simulink subsystem "VCM_main"  (R2021b)
settings: Solver=VariableStepAuto  StartTime=0.0  StopTime=10.0  RelTol=1e-3
values from neighbouring files (symbols this model uses):
  g = 9.80665    [VehicleParamsFEM20_Gear17.m]
  gear_f = 14.45    [VehicleParamsFEM20_Gear17.m]
  gear_r = 14.45    [VehicleParamsFEM20_Gear17.m]
  Iwf = 0.2    [VehicleParamsFEM20_Gear17.m]
  Rwf = 18*(25.4/1000)/2    (= 0.2286)    [VehicleParamsFEM20_Gear17.m]
libraries: simulink x46, dspswit3 x1, slpidlib x1
(part 3 of 5)

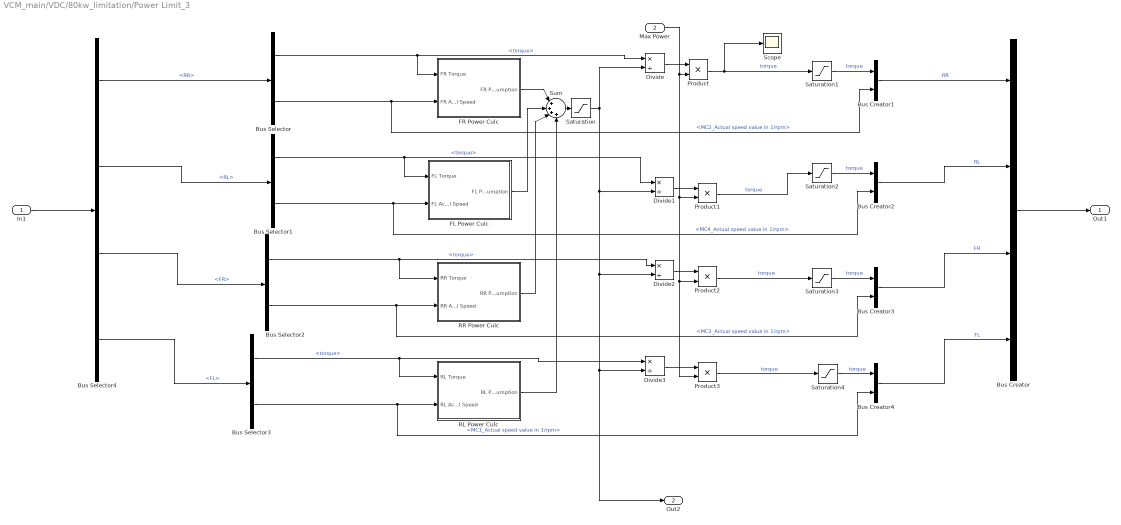
== system VCM_main/VDC/80kw_limitation/Power Limit_3 ==
  In1 : Inport
  Max Power : Inport  Port=2
  Bus Creator : BusCreator  Inputs=4
  Bus Creator{1..4} (4 alike) : BusCreator  Inputs=2
  Bus Selector : BusSelector  OutputSignals=torque,MC2_Actual speed value in 1/rpm
  Bus Selector1 : BusSelector  OutputSignals=torque,MC4_Actual speed value in 1/rpm
  Bus Selector2 : BusSelector  OutputSignals=torque,MC3_Actual speed value in 1/rpm
  Bus Selector3 : BusSelector  OutputSignals=torque,MC1_Actual speed value in 1/rpm
  Bus Selector4 : BusSelector  OutputSignals=RR,RL,FR,FL
  Divide{,1..3} (4 alike) : Product  Inputs=*/
  FL Power Culc : Subsystem
  FR Power Culc : Subsystem
  Product{,1..3} (4 alike) : Product
  RL Power Culc : Subsystem
  RR Power Culc : Subsystem
  Saturation : Saturate  UpperLimit=inf  LowerLimit=1
  Saturation{1..4} (4 alike) : Saturate  UpperLimit=21  LowerLimit=-21
  Scope : Scope
  Sum : Sum  Inputs=|++++
  Out1 : Outport  VectorParamsAs1DForOutWhenUnconnected=off
  Out2 : Outport  Port=2  VectorParamsAs1DForOutWhenUnconnected=off
  wires:
  Saturation4/1 -> Bus Creator4/1  "torque"
  Saturation3/1 -> Bus Creator3/1  "torque"
  Saturation2/1 -> Bus Creator2/1  "torque"
  Saturation1/1 -> Bus Creator1/1  "torque"
  Product1/1 -> Saturation2/1  "torque"
  Sum/1 -> Saturation/1
  Bus Creator4/1 -> Bus Creator/4  "FL"
  Product3/1 -> Saturation4/1  "torque"
  Bus Creator3/1 -> Bus Creator/3  "FR"
  Product2/1 -> Saturation3/1  "torque"
  Bus Creator2/1 -> Bus Creator/2  "RL"
  Bus Creator1/1 -> Bus Creator/1  "RR"
  Product/1 -> Saturation1/1, Scope/1  "torque"
  Bus Selector2/1 -> Divide2/1, RR Power Culc/1(RR Torque)  "<torque>"
  Bus Selector/1 -> FR Power Culc/1(FR Torque), Divide/1  "<torque>"
  Bus Selector1/2 -> Bus Creator2/2, FL Power Culc/2(FL Actual Speed)  "<MC4_Actual speed value in 1/rpm>"
  Bus Selector4/2 -> Bus Selector1/1  "<RL>"
  Saturation/1 -> Divide/2, Divide1/2, Divide2/2, Divide3/2, Out2/1
  Bus Selector3/1 -> RL Power Culc/1(RL Torque), Divide3/1  "<torque>"
  Bus Selector2/2 -> Bus Creator3/2, RR Power Culc/2(RR Actual Speed)  "<MC3_Actual speed value in 1/rpm>"
  Bus Selector1/1 -> FL Power Culc/1(FL Torque), Divide1/1  "<torque>"
  Bus Selector3/2 -> Bus Creator4/2, RL Power Culc/2(RL Actual Speed)  "<MC1_Actual speed value in 1/rpm>"
  RR Power Culc/1(RR Power Consumption) -> Sum/3
  RL Power Culc/1(RL Power Consumption) -> Sum/4
  Bus Selector4/1 -> Bus Selector/1  "<RR>"
  Divide/1 -> Product/1
  Divide1/1 -> Product1/1
  Bus Selector/2 -> Bus Creator1/2, FR Power Culc/2(FR Actual Speed)  "<MC2_Actual speed value in 1/rpm>"
  In1/1 -> Bus Selector4/1
  FR Power Culc/1(FR Power Consumption) -> Sum/1
  FL Power Culc/1(FL Power Consumption) -> Sum/2
  Bus Creator/1 -> Out1/1
  Bus Selector4/4 -> Bus Selector3/1  "<FL>"
  Bus Selector4/3 -> Bus Selector2/1  "<FR>"
  Divide3/1 -> Product3/1
  Divide2/1 -> Product2/1
  Max Power/1 -> Product/2, Product1/2, Product2/2, Product3/2

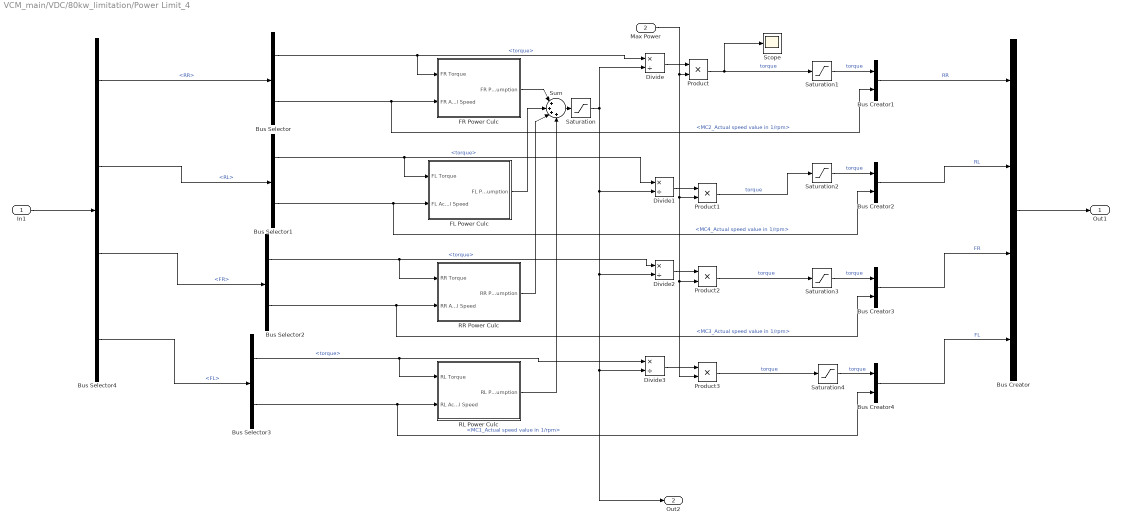
== system VCM_main/VDC/80kw_limitation/Power Limit_4 ==
  In1 : Inport
  Max Power : Inport  Port=2
  Bus Creator : BusCreator  Inputs=4
  Bus Creator{1..4} (4 alike) : BusCreator  Inputs=2
  Bus Selector : BusSelector  OutputSignals=torque,MC2_Actual speed value in 1/rpm
  Bus Selector1 : BusSelector  OutputSignals=torque,MC4_Actual speed value in 1/rpm
  Bus Selector2 : BusSelector  OutputSignals=torque,MC3_Actual speed value in 1/rpm
  Bus Selector3 : BusSelector  OutputSignals=torque,MC1_Actual speed value in 1/rpm
  Bus Selector4 : BusSelector  OutputSignals=RR,RL,FR,FL
  Divide{,1..3} (4 alike) : Product  Inputs=*/
  FL Power Culc : Subsystem
  FR Power Culc : Subsystem
  Product{,1..3} (4 alike) : Product
  RL Power Culc : Subsystem
  RR Power Culc : Subsystem
  Saturation : Saturate  UpperLimit=inf  LowerLimit=1
  Saturation{1..4} (4 alike) : Saturate  UpperLimit=21  LowerLimit=-21
  Scope : Scope
  Sum : Sum  Inputs=|++++
  Out1 : Outport  VectorParamsAs1DForOutWhenUnconnected=off
  Out2 : Outport  Port=2  VectorParamsAs1DForOutWhenUnconnected=off
  wires:
  Max Power/1 -> Product3/2, Product2/2, Product1/2, Product/2
  Divide2/1 -> Product2/1
  Divide3/1 -> Product3/1
  Bus Selector4/3 -> Bus Selector2/1  "<FR>"
  Bus Selector4/4 -> Bus Selector3/1  "<FL>"
  Bus Creator/1 -> Out1/1
  FL Power Culc/1(FL Power Consumption) -> Sum/2
  FR Power Culc/1(FR Power Consumption) -> Sum/1
  In1/1 -> Bus Selector4/1
  Bus Selector/2 -> FR Power Culc/2(FR Actual Speed), Bus Creator1/2  "<MC2_Actual speed value in 1/rpm>"
  Divide1/1 -> Product1/1
  Divide/1 -> Product/1
  Bus Selector4/1 -> Bus Selector/1  "<RR>"
  RL Power Culc/1(RL Power Consumption) -> Sum/4
  RR Power Culc/1(RR Power Consumption) -> Sum/3
  Bus Selector3/2 -> RL Power Culc/2(RL Actual Speed), Bus Creator4/2  "<MC1_Actual speed value in 1/rpm>"
  Bus Selector1/1 -> Divide1/1, FL Power Culc/1(FL Torque)  "<torque>"
  Bus Selector2/2 -> RR Power Culc/2(RR Actual Speed), Bus Creator3/2  "<MC3_Actual speed value in 1/rpm>"
  Bus Selector3/1 -> Divide3/1, RL Power Culc/1(RL Torque)  "<torque>"
  Saturation/1 -> Divide3/2, Out2/1, Divide2/2, Divide1/2, Divide/2
  Bus Selector4/2 -> Bus Selector1/1  "<RL>"
  Bus Selector1/2 -> FL Power Culc/2(FL Actual Speed), Bus Creator2/2  "<MC4_Actual speed value in 1/rpm>"
  Bus Selector/1 -> Divide/1, FR Power Culc/1(FR Torque)  "<torque>"
  Bus Selector2/1 -> RR Power Culc/1(RR Torque), Divide2/1  "<torque>"
  Product/1 -> Scope/1, Saturation1/1  "torque"
  Bus Creator1/1 -> Bus Creator/1  "RR"
  Bus Creator2/1 -> Bus Creator/2  "RL"
  Product2/1 -> Saturation3/1  "torque"
  Bus Creator3/1 -> Bus Creator/3  "FR"
  Product3/1 -> Saturation4/1  "torque"
  Bus Creator4/1 -> Bus Creator/4  "FL"
  Sum/1 -> Saturation/1
  Product1/1 -> Saturation2/1  "torque"
  Saturation1/1 -> Bus Creator1/1  "torque"
  Saturation2/1 -> Bus Creator2/1  "torque"
  Saturation3/1 -> Bus Creator3/1  "torque"
  Saturation4/1 -> Bus Creator4/1  "torque"

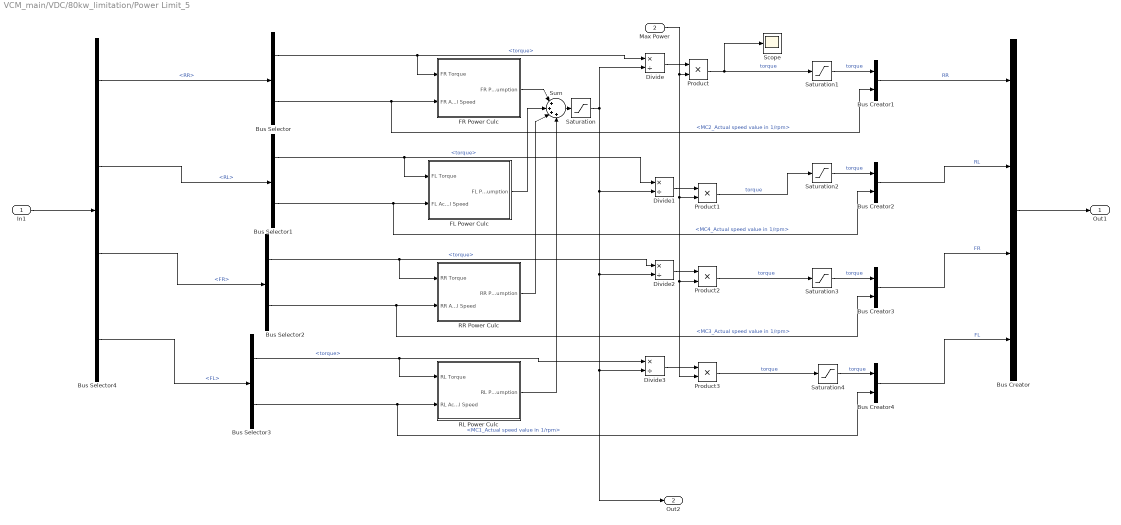
== system VCM_main/VDC/80kw_limitation/Power Limit_5 ==
  In1 : Inport
  Max Power : Inport  Port=2
  Bus Creator : BusCreator  Inputs=4
  Bus Creator{1..4} (4 alike) : BusCreator  Inputs=2
  Bus Selector : BusSelector  OutputSignals=torque,MC2_Actual speed value in 1/rpm
  Bus Selector1 : BusSelector  OutputSignals=torque,MC4_Actual speed value in 1/rpm
  Bus Selector2 : BusSelector  OutputSignals=torque,MC3_Actual speed value in 1/rpm
  Bus Selector3 : BusSelector  OutputSignals=torque,MC1_Actual speed value in 1/rpm
  Bus Selector4 : BusSelector  OutputSignals=RR,RL,FR,FL
  Divide{,1..3} (4 alike) : Product  Inputs=*/
  FL Power Culc : Subsystem
  FR Power Culc : Subsystem
  Product{,1..3} (4 alike) : Product
  RL Power Culc : Subsystem
  RR Power Culc : Subsystem
  Saturation : Saturate  UpperLimit=inf  LowerLimit=1
  Saturation{1..4} (4 alike) : Saturate  UpperLimit=21  LowerLimit=-21
  Scope : Scope
  Sum : Sum  Inputs=|++++
  Out1 : Outport  VectorParamsAs1DForOutWhenUnconnected=off
  Out2 : Outport  Port=2  VectorParamsAs1DForOutWhenUnconnected=off
  wires:
  Saturation4/1 -> Bus Creator4/1  "torque"
  Saturation3/1 -> Bus Creator3/1  "torque"
  Saturation2/1 -> Bus Creator2/1  "torque"
  Saturation1/1 -> Bus Creator1/1  "torque"
  Product1/1 -> Saturation2/1  "torque"
  Sum/1 -> Saturation/1
  Bus Creator4/1 -> Bus Creator/4  "FL"
  Product3/1 -> Saturation4/1  "torque"
  Bus Creator3/1 -> Bus Creator/3  "FR"
  Product2/1 -> Saturation3/1  "torque"
  Bus Creator2/1 -> Bus Creator/2  "RL"
  Bus Creator1/1 -> Bus Creator/1  "RR"
  Product/1 -> Saturation1/1, Scope/1  "torque"
  Bus Selector2/1 -> Divide2/1, RR Power Culc/1(RR Torque)  "<torque>"
  Bus Selector/1 -> FR Power Culc/1(FR Torque), Divide/1  "<torque>"
  Bus Selector1/2 -> Bus Creator2/2, FL Power Culc/2(FL Actual Speed)  "<MC4_Actual speed value in 1/rpm>"
  Bus Selector4/2 -> Bus Selector1/1  "<RL>"
  Saturation/1 -> Divide/2, Divide1/2, Divide2/2, Divide3/2, Out2/1
  Bus Selector3/1 -> RL Power Culc/1(RL Torque), Divide3/1  "<torque>"
  Bus Selector2/2 -> Bus Creator3/2, RR Power Culc/2(RR Actual Speed)  "<MC3_Actual speed value in 1/rpm>"
  Bus Selector1/1 -> FL Power Culc/1(FL Torque), Divide1/1  "<torque>"
  Bus Selector3/2 -> Bus Creator4/2, RL Power Culc/2(RL Actual Speed)  "<MC1_Actual speed value in 1/rpm>"
  RR Power Culc/1(RR Power Consumption) -> Sum/3
  RL Power Culc/1(RL Power Consumption) -> Sum/4
  Bus Selector4/1 -> Bus Selector/1  "<RR>"
  Divide/1 -> Product/1
  Divide1/1 -> Product1/1
  Bus Selector/2 -> Bus Creator1/2, FR Power Culc/2(FR Actual Speed)  "<MC2_Actual speed value in 1/rpm>"
  In1/1 -> Bus Selector4/1
  FR Power Culc/1(FR Power Consumption) -> Sum/1
  FL Power Culc/1(FL Power Consumption) -> Sum/2
  Bus Creator/1 -> Out1/1
  Bus Selector4/4 -> Bus Selector3/1  "<FL>"
  Bus Selector4/3 -> Bus Selector2/1  "<FR>"
  Divide3/1 -> Product3/1
  Divide2/1 -> Product2/1
  Max Power/1 -> Product/2, Product1/2, Product2/2, Product3/2

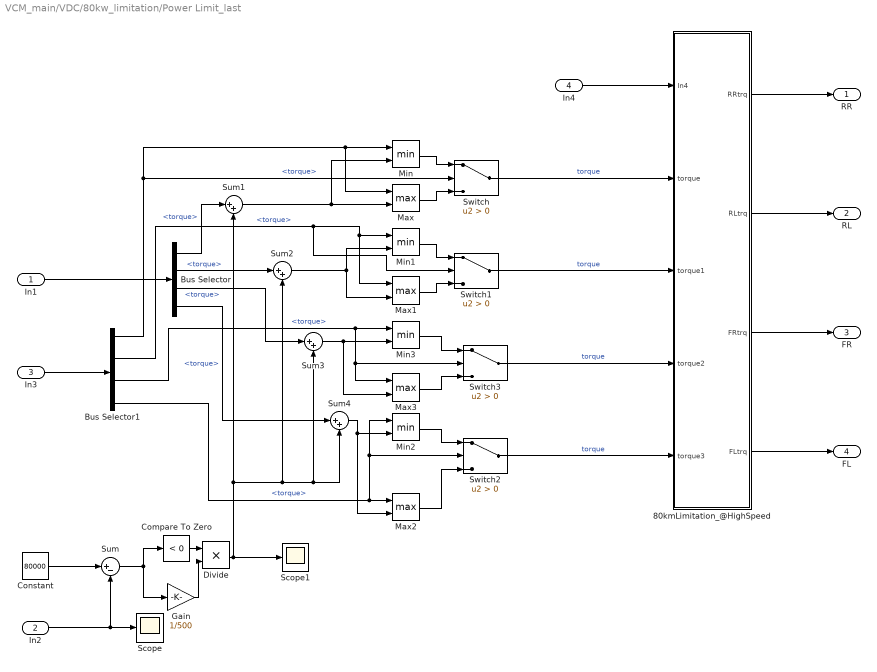
== system VCM_main/VDC/80kw_limitation/Power Limit_last ==
  In1 : Inport
  In2 : Inport  Port=2
  In3 : Inport  Port=3
  In4 : Inport  Port=4
  80kmLimitation_@HighSpeed : Subsystem
  Bus Selector : BusSelector  OutputSignals=RR.torque,RL.torque,FR.torque,FL.torque
  Bus Selector1 : BusSelector  OutputSignals=RR.torque,RL.torque,FR.torque,FL.torque
  Compare To Zero : simulink/Logic and Bit Operations/Compare To Zero  relop=<  OutDataTypeStr=boolean
  Constant : Constant  Value=80000
  Divide : Product  Inputs=**
  Gain : Gain  Gain=1/500
  Max{,1..3} (4 alike) : MinMax  Function=max  Inputs=2
  Min{,1..3} (4 alike) : MinMax  Inputs=2
  Scope : Scope
  Scope1 : Scope
  Sum : Sum  Inputs=|+-
  Sum{1..4} (4 alike) : Sum  Inputs=|++
  Switch{,1..3} (4 alike) : Switch  Criteria=u2 > Threshold
  RR : Outport  VectorParamsAs1DForOutWhenUnconnected=off
  RL : Outport  Port=2  VectorParamsAs1DForOutWhenUnconnected=off
  FR : Outport  Port=3  VectorParamsAs1DForOutWhenUnconnected=off
  FL : Outport  Port=4  VectorParamsAs1DForOutWhenUnconnected=off
  wires:
  Gain/1 -> Divide/2
  Compare To Zero/1 -> Divide/1
  80kmLimitation_@HighSpeed/4(FLtrq) -> FL/1
  80kmLimitation_@HighSpeed/2(RLtrq) -> RL/1
  80kmLimitation_@HighSpeed/3(FRtrq) -> FR/1
  80kmLimitation_@HighSpeed/1(RRtrq) -> RR/1
  Switch2/1 -> 80kmLimitation_@HighSpeed/5(torque3)  "torque"
  Switch3/1 -> 80kmLimitation_@HighSpeed/4(torque2)  "torque"
  Switch1/1 -> 80kmLimitation_@HighSpeed/3(torque1)  "torque"
  Switch/1 -> 80kmLimitation_@HighSpeed/2(torque)  "torque"
  In4/1 -> 80kmLimitation_@HighSpeed/1(In4)
  Max3/1 -> Switch3/3
  Min3/1 -> Switch3/1
  Max2/1 -> Switch2/3
  Min2/1 -> Switch2/1
  Max1/1 -> Switch1/3
  Min1/1 -> Switch1/1
  Max/1 -> Switch/3
  Min/1 -> Switch/1
  Bus Selector1/4 -> Max2/1, Switch2/2, Min2/1  "<torque>"
  Sum4/1 -> Min2/2, Max2/2
  Bus Selector1/3 -> Min3/1, Switch3/2, Max3/1  "<torque>"
  Sum3/1 -> Min3/2, Max3/2
  Bus Selector1/2 -> Min1/1, Max1/1, Switch1/2  "<torque>"
  Sum2/1 -> Min1/2, Max1/2
  Bus Selector1/1 -> Max/1, Min/1, Switch/2  "<torque>"
  Sum1/1 -> Min/2, Max/2
  In3/1 -> Bus Selector1/1
  Bus Selector/4 -> Sum4/1  "<torque>"
  Bus Selector/3 -> Sum3/1  "<torque>"
  Bus Selector/2 -> Sum2/1  "<torque>"
  Divide/1 -> Scope1/1, Sum3/2, Sum4/2, Sum2/2, Sum1/2
  Bus Selector/1 -> Sum1/1  "<torque>"
  In1/1 -> Bus Selector/1
  Sum/1 -> Gain/1, Compare To Zero/1
  In2/1 -> Scope/1, Sum/2
  Constant/1 -> Sum/1

== system VCM_main/VDC/80kw_limitation/Subsystem ==
  In1 : Inport
  RR : Inport  Port=2
  RL : Inport  Port=3
  FR : Inport  Port=4
  FL : Inport  Port=5
  Bus Creator : BusCreator  Inputs=4
  Bus Selector : BusSelector  OutputSignals=RR.torque,RL.torque,FR.torque,FL.torque
  Switch{,1..3} (4 alike) : Switch  Criteria=u2 > Threshold  Threshold=0.5
  Out1 : Outport  VectorParamsAs1DForOutWhenUnconnected=off
  wires:
  RL/1 -> Switch1/1
  RR/1 -> Switch/1
  In1/1 -> Bus Selector/1
  FR/1 -> Switch2/1
  Bus Selector/2 -> Switch1/3  "<torque>"
  Switch3/1 -> Bus Creator/4  "FLtorque"
  Switch1/1 -> Bus Creator/2  "RLtorque"
  Bus Creator/1 -> Out1/1
  Bus Selector/4 -> Switch3/3  "<torque>"
  Switch/1 -> Bus Creator/1  "RRtorque"
  FL/1 -> Switch3/1
  Switch2/1 -> Bus Creator/3  "FRtorque"
  Bus Selector/1 -> Switch/3  "<torque>"
  [PowerLimitOn] -> Switch1/2, Switch/2, Switch2/2, Switch3/2
  Bus Selector/3 -> Switch2/3  "<torque>"

== system VCM_main/VDC/DYC/Moment to ΔT ==
  TargetYawMoment : Inport
  Gain12 : Gain  Gain=1/4
  Gain13 : Gain  Gain=1/0.625
  Gain14 : Gain  Gain=1/13.75
  Gain4 : Gain  Gain=18*(25.4/1000)/2
  Saturation : Saturate  UpperLimit=5  LowerLimit=-5
  DYC_deltaTorque : Outport
  wires:
  Saturation/1 -> DYC_deltaTorque/1  "DYC_deltaTorque"
  Gain4/1 -> Saturation/1
  Gain14/1 -> Gain4/1
  Gain12/1 -> Gain13/1
  TargetYawMoment/1 -> Gain12/1
  Gain13/1 -> Gain14/1

== system VCM_main/VDC/DYC/Torque distributor1 ==
  Torque In : Inport
  In2 : Inport  Port=2
  Add : Sum
  Logical Operator : Logic  AllPortsSameDT=off  OutDataTypeStr=boolean
  Switch : Switch  Criteria=u2 > Threshold  Threshold=0.5
  torque : Outport
  wires:
  Logical Operator/1 -> Switch/2
  [All_bQuitInverterOn] -> Logical Operator/2
  Switch/1 -> torque/1
  [DYCOn] -> Logical Operator/1
  In2/1 -> Add/2
  Add/1 -> Switch/1  "torque"
  Torque In/1 -> Add/1, Switch/3

== system VCM_main/VDC/DYC/Torque distributor2 ==
  Torque In : Inport
  In2 : Inport  Port=2
  Add : Sum
  Logical Operator : Logic  AllPortsSameDT=off  OutDataTypeStr=boolean
  Switch : Switch  Criteria=u2 > Threshold  Threshold=0.5
  torque : Outport
  wires:
  Torque In/1 -> Switch/3, Add/1
  Add/1 -> Switch/1  "torque"
  In2/1 -> Add/2
  [DYCOn] -> Logical Operator/1
  Switch/1 -> torque/1
  [All_bQuitInverterOn] -> Logical Operator/2
  Logical Operator/1 -> Switch/2

== system VCM_main/VDC/DYC/Torque distributor3 ==
  Torque In : Inport
  In2 : Inport  Port=2
  Add : Sum
  Logical Operator : Logic  AllPortsSameDT=off  OutDataTypeStr=boolean
  Switch : Switch  Criteria=u2 > Threshold  Threshold=0.5
  torque : Outport
  wires:
  Logical Operator/1 -> Switch/2
  [All_bQuitInverterOn] -> Logical Operator/2
  Switch/1 -> torque/1
  [DYCOn] -> Logical Operator/1
  In2/1 -> Add/2
  Add/1 -> Switch/1  "torque"
  Torque In/1 -> Add/1, Switch/3

== system VCM_main/VDC/DYC/Torque distributor4 ==
  Torque In : Inport
  DYC_deltaTorque : Inport  Port=2
  Add : Sum
  Logical Operator : Logic  AllPortsSameDT=off  OutDataTypeStr=boolean
  Switch : Switch  Criteria=u2 > Threshold  Threshold=0.5
  torque : Outport
  wires:
  Torque In/1 -> Switch/3, Add/1
  Add/1 -> Switch/1  "torque"
  DYC_deltaTorque/1 -> Add/2
  [DYCOn] -> Logical Operator/1
  Switch/1 -> torque/1
  [All_bQuitInverterOn] -> Logical Operator/2
  Logical Operator/1 -> Switch/2

== system VCM_main/VDC/DYC/YawmomentCal ==
  DriverInput : Inport
  Sensor : Inport  Port=2
  Bus Selector1 : BusSelector  OutputSignals=CAN_from_IMU_122.GYRO_Z,CAN_from_IMU_220.ANGLE_SLIP
  Bus Selector2 : BusSelector  OutputSignals=SteerAngle_Actual
  FB : Subsystem
  FF_Gain : Subsystem
  FF_diff_Gain : Subsystem
  Gain : Gain  Gain=300
  Ground : Ground
  Scope : Scope
  Sensor1 : InportShadow  Port=2
  StabilityFactor_ref : Constant  Value=0.00125
  Sum : Sum  Inputs=|++
  Sum1 : Sum  Inputs=|++
  Sum2 : Sum  Inputs=|-+
  Terminator : Terminator
  Terminator1 : Terminator
  Terminator3 : Terminator
  Velocity Clc : Subsystem
  stabilityfactor_noDYC : Constant  Value=0.00604
  δ to r_noDYC : Subsystem
  δ to r_ref : Subsystem
  TargetYawMoment : Outport  VectorParamsAs1DForOutWhenUnconnected=off
  r_ref : Outport  Port=2
  wires:
  Sum1/1 -> Terminator3/1
  FB/1(y) -> Sum1/2
  Ground/1 -> Sum/2
  Bus Selector1/1 -> FB/2(<GYRO_Z>)  "<GYRO_Z>"
  Sum/1 -> Sum1/1
  FF_diff_Gain/1(Out1) -> Terminator/1
  FF_Gain/1(Out1) -> Sum/1
  Velocity Clc/1(v [m/s]) -> δ to r_ref/1(v [m/s]), δ to r_noDYC/1(v [m/s]), FF_Gain/1(v [m/s]), FF_diff_Gain/1(v [m/s])
  Sensor/1 -> Velocity Clc/1(Sensor)
  Bus Selector1/2 -> Terminator1/1  "<ANGLE_SLIP>"
  Sensor1/1 -> Bus Selector1/1
  Sum2/1 -> FF_Gain/2(In1), FF_diff_Gain/2(In2), Scope/1
  Gain/1 -> TargetYawMoment/1  "TargetYawMoment"
  δ to r_noDYC/1(r_noDYC) -> Sum2/1  "r_noDYC"
  stabilityfactor_noDYC/1 -> δ to r_noDYC/2(StabilityFactor)
  Bus Selector2/1 -> δ to r_noDYC/3(SteerAngle), δ to r_ref/3(SteerAngle), Gain/1  "<SteerAngle_Actual>"
  DriverInput/1 -> Bus Selector2/1
  δ to r_ref/1(r_ref) -> Sum2/2, FB/1(r_ref), r_ref/1  "r_ref"
  StabilityFactor_ref/1 -> δ to r_ref/2(StabilityFactor)

== system VCM_main/VDC/Launch/max rpm ==
  Can Inv : Inport
  Bus Selector4 : BusSelector  OutputSignals=MC_11.MC1_Actual speed value in 1/rpm,MC_31.MC3_Actual speed value in 1/rpm,MC_21.MC2_Actual speed value in 1/rpm,MC_41.MC4_Actual speed value in 1/rpm
  Min : MinMax  Function=max  Inputs=4
  max rpm : Outport
  wires:
  Bus Selector4/2 -> Min/2  "<MC3_Actual speed value in 1/rpm>"
  Bus Selector4/3 -> Min/3  "<MC2_Actual speed value in 1/rpm>"
  Bus Selector4/1 -> Min/1  "<MC1_Actual speed value in 1/rpm>"
  Min/1 -> max rpm/1  "max rpm"
  Can Inv/1 -> Bus Selector4/1
  Bus Selector4/4 -> Min/4  "<MC4_Actual speed value in 1/rpm>"

== system VCM_main/VDC/Torque Front//rear distributor Main/Max Torque Limit ==
  note: MAXトルクオーバーしている分だけもう一方に振り直し
  Max Torque : Inport
  torque_front : Inport  Port=2
  torque_rear : Inport  Port=3
  Add10 : Sum  Inputs=-+
  Add11 : Sum
  Add4 : Sum  Inputs=+-
  Add7 : Sum  Inputs=+-
  Add8 : Sum
  Add9 : Sum  Inputs=+-
  Display : Display
  Display5 : Display
  Display6 : Display
  Saturation : Saturate  UpperLimit=inf  LowerLimit=0
  Saturation3 : Saturate  UpperLimit=inf  LowerLimit=0
  torque_front Out : Outport
  torque_rear Out : Outport  Port=2
  wires:
  Max Torque/1 -> Add9/2, Add4/2
  Add11/1 -> torque_rear Out/1
  Add7/1 -> Add11/2
  Add4/1 -> Saturation/1
  Add10/1 -> torque_front Out/1
  Add8/1 -> Add10/2
  torque_rear/1 -> Display6/1, Add7/1, Add4/1
  Add9/1 -> Saturation3/1
  torque_front/1 -> Display5/1, Add8/1, Add9/1
  Saturation3/1 -> Add10/1, Add11/1
  Saturation/1 -> Display/1, Add7/2, Add8/2

== system VCM_main/VDC/Torque Front//rear distributor Main/Min Torque Limit ==
  note: MINトルクオーバーしている分だけもう一方に振り直し
  Min Torque : Inport
  torque_front : Inport  Port=2
  torque_rear : Inport  Port=3
  Add10 : Sum  Inputs=-+
  Add11 : Sum
  Add4 : Sum  Inputs=+-
  Add7 : Sum  Inputs=+-
  Add8 : Sum
  Add9 : Sum  Inputs=+-
  Display{,1..2,5..6} (5 alike) : Display
  Gain : Gain  Gain=-1
  Saturation : Saturate  UpperLimit=0  LowerLimit=-inf
  Saturation3 : Saturate  UpperLimit=0  LowerLimit=-inf
  torque_rear Out : Outport
  torque_front Out : Outport  Port=2
  wires:
  Gain/1 -> Add9/2, Add4/2
  Min Torque/1 -> Gain/1
  Add11/1 -> torque_rear Out/1  "torque_rear"
  Add7/1 -> Add11/2, Display1/1
  Add4/1 -> Saturation/1
  Add10/1 -> torque_front Out/1  "torque_front"
  Add8/1 -> Add10/2
  torque_rear/1 -> Display6/1, Add7/1, Add4/1
  Add9/1 -> Saturation3/1
  torque_front/1 -> Display5/1, Add8/1, Add9/1
  Saturation3/1 -> Add10/1, Add11/1, Display2/1
  Saturation/1 -> Display/1, Add7/2, Add8/2

== system VCM_main/VDC/Torque Front//rear distributor Main/Saturation ==
  u : Inport
  Saturation Dynamic1 : simulink/Discontinuities/Saturation Dynamic  OutMin=[]  OutMax=[]  OutDataTypeStr=Inherit: Same as second input  OutDataType=fixdt(1, 16)  OutScaling=2^-10  DoSatur=off
  y : Outport
  wires:
  u/1 -> Saturation Dynamic1/2
  Saturation Dynamic1/1 -> y/1
  [MinTorque] -> Saturation Dynamic1/3
  [MaxTorque] -> Saturation Dynamic1/1

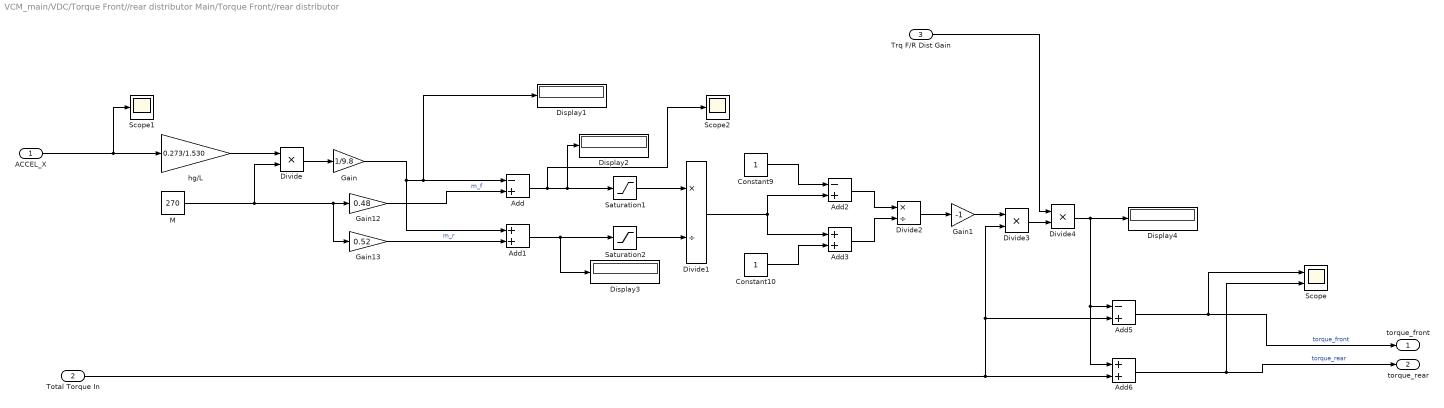
== system VCM_main/VDC/Torque Front//rear distributor Main/Torque Front//rear distributor  ==
  ACCEL_X : Inport
  Total Torque In : Inport  Port=2
  Trq F/R Dist Gain : Inport  Port=3
  Add : Sum  Inputs=-+
  Add1 : Sum
  Add2 : Sum  Inputs=-+
  Add3 : Sum
  Add5 : Sum  Inputs=-+
  Add6 : Sum
  Constant10 : Constant
  Constant9 : Constant
  Display{1..4} (4 alike) : Display
  Divide : Product  Inputs=**
  Divide1 : Product  Inputs=*/
  Divide2 : Product  Inputs=*/
  Divide3 : Product  Inputs=**
  Divide4 : Product  Inputs=**
  Gain : Gain  Gain=1/9.8
  Gain1 : Gain  Gain=-1
  Gain12 : Gain  Gain=0.48
  Gain13 : Gain  Gain=0.52
  M : Constant  Value=270
  Saturation1 : Saturate  UpperLimit=270  LowerLimit=10
  Saturation2 : Saturate  UpperLimit=270  LowerLimit=10
  Scope : Scope  NumInputPorts=2
  Scope1 : Scope
  Scope2 : Scope
  hg/L : Gain  Gain=0.273/1.530
  torque_front : Outport
  torque_rear : Outport  Port=2
  wires:
  Divide/1 -> Gain/1
  Total Torque In/1 -> Divide3/2, Add5/2, Add6/2
  Trq F/R Dist Gain/1 -> Divide4/1
  Divide3/1 -> Divide4/2
  Add5/1 -> torque_front/1, Scope/1  "torque_front"
  Add6/1 -> torque_rear/1, Scope/2  "torque_rear"
  Gain13/1 -> Add1/2  "m_r"
  Saturation1/1 -> Divide1/1
  Add/1 -> Saturation1/1, Display2/1, Scope2/1
  Gain/1 -> Add/1, Display1/1, Add1/1
  Add1/1 -> Saturation2/1, Display3/1
  ACCEL_X/1 -> hg/L/1, Scope1/1
  hg/L/1 -> Divide/1
  Constant10/1 -> Add3/2
  Gain1/1 -> Divide3/1
  Add2/1 -> Divide2/1
  Gain12/1 -> Add/2  "m_f"
  Divide2/1 -> Gain1/1
  Constant9/1 -> Add2/1
  Saturation2/1 -> Divide1/2
  Divide4/1 -> Display4/1, Add5/1, Add6/1
  Add3/1 -> Divide2/2
  Divide1/1 -> Add2/2, Add3/1
  M/1 -> Gain12/1, Gain13/1, Divide/2

== system VCM_main/VDC/Traction Control/FF ==
  note: FEM20
      | ４駆21Nmなら1.25G
      | ４駆10Nmなら1G
  target speed : Inport
  1/ tire R1 : Gain  Gain=1/Rwf
  1/(1-SlipRate) : Subsystem
  1/Gear : Gain  Gain=1/gear_f
  1/Gear1 : Gain  Gain=1/gear_f
  1/Gear2 : Gain  Gain=1/gear_r
  Add : Sum
  Add1 : Sum
  Add2 : Sum
  FF : Scope  NumInputPorts=4
  FR Load Diff : Subsystem  ReferencedSubsystem=FR_Load_Diff
  Fd : Lookup_n-D  NumberOfTableDimensions=1  BreakpointsForDimension1=|  Table=|  InternalRulePriority=Speed  RndMeth=Simplest  InputSameDT=on
      BreakpointsForDimension1=|
      | [2430
      | 3385
      | 4780
      | 5950
      | 7650
      | 10810
      | 13260
      | 15350
      | 17190]
      Table=|
      | [0.55
      | 0.6
      | 0.7
      | 0.8
      | 1
      | 1.5
      | 2
      | 2.5
      | 3]
  Rtire : Gain  Gain=Rwf
  Rtire1 : Gain  Gain=1/gear_r
  Target Acc : Constant  Value=1*g
  Target SlipRate : Constant  Value=0.18
  Tire Force F : Subsystem  ReferencedSubsystem=Tire_Force
  Tire Force F1 : Subsystem  ReferencedSubsystem=Tire_Force
  wheel Inertia : Gain  Gain=Iwf
  FF_R : Outport
  FF_F : Outport  Port=2
  wires:
  Rtire1/1 -> 1/Gear2/1
  1/Gear2/1 -> FF/4, Add2/2  "r*F Rr"
  1/Gear1/1 -> Add1/2, FF/3  "r*F Fr"
  wheel Inertia/1 -> 1/Gear/1
  1/ tire R1/1 -> wheel Inertia/1  "omega'"
  1/Gear/1 -> FF/2, Add/2  "I*omega'"
  Fd/1 -> Add/1, FF/1  "T_loss"
  Add1/1 -> FF_F/1
  Rtire/1 -> 1/Gear1/1
  target speed/1 -> Fd/1
  Add/1 -> Add1/1, Add2/1
  Add2/1 -> FF_R/1
  Tire Force F/1 -> Rtire1/1
  FR Load Diff/1 -> Tire Force F1/1
  FR Load Diff/2 -> Tire Force F/1
  Tire Force F1/1 -> Rtire/1
  Target SlipRate/1 -> 1/(1-SlipRate)/2(SlipRate), Tire Force F/2, Tire Force F1/2
  1/(1-SlipRate)/1(Out) -> 1/ tire R1/1  "V_wheel'"
  Target Acc/1 -> 1/(1-SlipRate)/1(In), FR Load Diff/1

== system VCM_main/VDC/Traction Control/Front TargetSpeedClc_inBrake ==
  SensorIn : Inport
  Bus Selector : BusSelector  OutputSignals=CAN_from_IMU_139.VELOCITY_X
  Constant : Constant  Value=0
  Front sliprate_inBrake_ref : Constant  Value=0.18
  FrontGain : Gain  Gain=1.2
  Gear : Gain  Gain=13.75
  Saturation Dynamic : simulink/Discontinuities/Saturation Dynamic  OutMin=[]  OutMax=[]  OutDataTypeStr=Inherit: Same as second input  OutDataType=fixdt(1, 16)  OutScaling=2^-10  DoSatur=off
  Scope : Scope
  toTargetspeed : Subsystem
  toTire_rpm : Gain  Gain=60/(2*pi*0.228)
  target speed : Outport  VectorParamsAs1DForOutWhenUnconnected=off
  wires:
  Front sliprate_inBrake_ref/1 -> toTargetspeed/1(In1)
  FrontGain/1 -> Saturation Dynamic/2, Scope/1
  SensorIn/1 -> Bus Selector/1
  [speedlimit] -> Saturation Dynamic/1
  toTargetspeed/1(Out1) -> FrontGain/1
  Bus Selector/1 -> toTire_rpm/1  "<VELOCITY_X>"
  Constant/1 -> Saturation Dynamic/3
  Gear/1 -> toTargetspeed/2(In2)
  Saturation Dynamic/1 -> target speed/1  "target speed"
  toTire_rpm/1 -> Gear/1

== system VCM_main/VDC/Traction Control/Rear TargetSpeedClc_inBrake ==
  SensorIn : Inport
  Bus Selector : BusSelector  OutputSignals=CAN_from_IMU_139.VELOCITY_X
  Constant : Constant  Value=0
  Gear : Gain  Gain=13.75
  Rear sliprate_inBrake_ref : Constant  Value=0.18
  Saturation Dynamic : simulink/Discontinuities/Saturation Dynamic  OutMin=[]  OutMax=[]  OutDataTypeStr=Inherit: Same as second input  OutDataType=fixdt(1, 16)  OutScaling=2^-10  DoSatur=off
  toTargetspeed : Subsystem
  toTire_rpm : Gain  Gain=60/(2*pi*0.228)
  target speed : Outport  VectorParamsAs1DForOutWhenUnconnected=off
  wires:
  Rear sliprate_inBrake_ref/1 -> toTargetspeed/1(In1)
  toTire_rpm/1 -> Gear/1
  Saturation Dynamic/1 -> target speed/1  "target speed"
  Gear/1 -> toTargetspeed/2(In2)
  Constant/1 -> Saturation Dynamic/3
  Bus Selector/1 -> toTire_rpm/1  "<VELOCITY_X>"
  toTargetspeed/1(Out1) -> Saturation Dynamic/2
  [speedlimit] -> Saturation Dynamic/1
  SensorIn/1 -> Bus Selector/1

== system VCM_main/VDC/Traction Control/TargetSpeed_inAcc ==
  note: 速度センサの遅れ補償
  Torque In : Inport
  SensorIn : Inport  Port=2
  Add : Sum
  Bus Selector : BusSelector  OutputSignals=CAN_from_IMU_139.VELOCITY_X
  Bus Selector1 : BusSelector  OutputSignals=RRtorque,RLtorque,FRtorque,FLtorque
  Compare To Zero{,1..3} (4 alike) : simulink/Logic and Bit Operations/Compare To Zero  relop===  OutDataTypeStr=boolean
  Constant : Constant  Value=100
  Constant1 : Constant  Value=1*g*0.001
  Constant2 : Constant  Value=0
  Gear : Gain  Gain=gear_f
  Logical Operator : Logic  Inputs=4  AllPortsSameDT=off  OutDataTypeStr=boolean
  Logical Operator1 : Logic  Operator=NOT  AllPortsSameDT=off  OutDataTypeStr=boolean
  Product : Product
  Rear_sliprate_ref : Constant  Value=0.18
  Saturation Dynamic : simulink/Discontinuities/Saturation Dynamic  OutMin=[]  OutMax=[]  OutDataTypeStr=Inherit: Same as second input  OutDataType=fixdt(1, 16)  OutScaling=2^-10  DoSatur=off
  Scope : Scope
  Scope1 : Scope
  Sqrt : Sqrt  SaturateOnIntegerOverflow=on
  Switch : Switch  Criteria=u2 > Threshold
  Time msec : Gain  Gain=80
  toTargetspeed : Subsystem
  toTire_rpm : Gain  Gain=60/(2*pi*Rwf)
  target speed : Outport  VectorParamsAs1DForOutWhenUnconnected=off
  wires:
  Add/1 -> toTire_rpm/1
  Time msec/1 -> Add/2
  Constant1/1 -> Time msec/1
  Sqrt/1 -> Add/1
  Product/1 -> Sqrt/1
  Rear_sliprate_ref/1 -> toTargetspeed/1(In1)
  SensorIn/1 -> Bus Selector/1
  [speedlimit] -> Saturation Dynamic/1
  Gear/1 -> Saturation Dynamic/2, Scope1/1
  Bus Selector/1 -> Product/1, Product/2  "<VELOCITY_X>"
  Constant/1 -> Saturation Dynamic/3
  Saturation Dynamic/1 -> toTargetspeed/2(y)  "target speed"
  toTire_rpm/1 -> Gear/1
  Torque In/1 -> Bus Selector1/1
  Bus Selector1/2 -> Compare To Zero1/1  "<RLtorque>"
  Bus Selector1/3 -> Compare To Zero2/1  "<FRtorque>"
  Bus Selector1/4 -> Compare To Zero3/1  "<FLtorque>"
  Bus Selector1/1 -> Compare To Zero/1  "<RRtorque>"
  Compare To Zero/1 -> Logical Operator/1
  Compare To Zero1/1 -> Logical Operator/2
  Compare To Zero2/1 -> Logical Operator/3
  Compare To Zero3/1 -> Logical Operator/4
  Constant2/1 -> Switch/3
  Logical Operator/1 -> Logical Operator1/1
  Logical Operator1/1 -> Switch/2
  toTargetspeed/1(Out1) -> Switch/1
  Switch/1 -> Scope/1, target speed/1

== system VCM_main/VDC/VCM_Status/Sliprate ==
  In1 : Inport
  In2 : Inport  Port=2
  Bus Creator : BusCreator  Inputs=4
  Bus Selector1 : BusSelector  OutputSignals=MC_41.MC4_Actual speed value in 1/rpm,MC_21.MC2_Actual speed value in 1/rpm,MC_31.MC3_Actual speed value in 1/rpm,MC_11.MC1_Actual speed value in 1/rpm
  Bus Selector4 : BusSelector  OutputSignals=CAN_from_IMU_139.VELOCITY_X
  Scope : Scope  NumInputPorts=4
  Sliprate Calculator : Subsystem
  Sliprate : Outport
  wires:
  Bus Creator/1 -> Sliprate/1  "Sliprate"
  In2/1 -> Bus Selector1/1
  In1/1 -> Bus Selector4/1
  Sliprate Calculator/1(FL_Sliprate) -> Bus Creator/1, Scope/1
  Sliprate Calculator/4(FR_Sliprate) -> Bus Creator/4, Scope/4
  Sliprate Calculator/2(RR_Sliprate) -> Bus Creator/2, Scope/2
  Sliprate Calculator/3(RL_Sliprate) -> Bus Creator/3, Scope/3
  Bus Selector1/1 -> Sliprate Calculator/2(<MC4_Actual speed value in 1/rpm>)  "<MC4_Actual speed value in 1/rpm>"
  Bus Selector4/1 -> Sliprate Calculator/1(<VELOCITY_X>)  "<VELOCITY_X>"
  Bus Selector1/4 -> Sliprate Calculator/5(<MC1_Actual speed value in 1/rpm>)  "<MC1_Actual speed value in 1/rpm>"
  Bus Selector1/2 -> Sliprate Calculator/3(<MC2_Actual speed value in 1/rpm>)  "<MC2_Actual speed value in 1/rpm>"
  Bus Selector1/3 -> Sliprate Calculator/4(<MC3_Actual speed value in 1/rpm>)  "<MC3_Actual speed value in 1/rpm>"

== system VCM_main/VDC/VCM_Status/VCMStatus_bus ==
  In1 : Inport
  Bus Creator1 : BusCreator  Inputs=7
  Logical Operator1 : Logic  AllPortsSameDT=off  OutDataTypeStr=boolean
  VCMStatus : Outport
  wires:
  Bus Creator1/1 -> VCMStatus/1  "VCMStatus"
  In1/1 -> Logical Operator1/1
  [PowerLimitOn] -> Bus Creator1/7  "80kWOn"
  [TCOn] -> Bus Creator1/4  "TCOn"
  Logical Operator1/1 -> Bus Creator1/1  "VDCStatus"
  [VDCOn] -> Logical Operator1/2
  [DYCOn] -> Bus Creator1/6  "DYCOn"
  [ABSOn] -> Bus Creator1/5  "ABSOn"
  [BrakeOverRide] -> Bus Creator1/3  "BrakeOverRide"
  [APPS_SafetyError] -> Bus Creator1/2  "APPS_SafetyError"

== system VCM_main/Error display Box/Error Info/error memory MC1/Triggered Subsystem ==
  In1 : Inport
  Trigger : TriggerPort  VariantControl=Variant
  Delay : Delay  DelayLength=1  InitialCondition=0
  Delay1 : Delay  InitialCondition=0
  Out1 : Outport  VectorParamsAs1DForOutWhenUnconnected=off
  Out2 : Outport  Port=2  InitialOutput=[0]  VectorParamsAs1DForOutWhenUnconnected=off
  Out3 : Outport  Port=3  InitialOutput=[0]  VectorParamsAs1DForOutWhenUnconnected=off
  wires:
  Delay1/1 -> Out3/1
  Delay/1 -> Out2/1
  In1/1 -> Out1/1, Delay1/1, Delay/1

== system VCM_main/Error display Box/Error Info/error memory MC2/Triggered Subsystem ==
  In1 : Inport
  Trigger : TriggerPort  VariantControl=Variant
  Delay : Delay  DelayLength=1  InitialCondition=0
  Delay1 : Delay  InitialCondition=0
  Out1 : Outport  VectorParamsAs1DForOutWhenUnconnected=off
  Out2 : Outport  Port=2  InitialOutput=[0]  VectorParamsAs1DForOutWhenUnconnected=off
  Out3 : Outport  Port=3  InitialOutput=[0]  VectorParamsAs1DForOutWhenUnconnected=off
  wires:
  Delay1/1 -> Out3/1
  Delay/1 -> Out2/1
  In1/1 -> Out1/1, Delay1/1, Delay/1

== system VCM_main/Error display Box/Error Info/error memory MC3/Triggered Subsystem ==
  In1 : Inport
  Trigger : TriggerPort  VariantControl=Variant
  Delay : Delay  DelayLength=1  InitialCondition=0
  Delay1 : Delay  InitialCondition=0
  Out1 : Outport  VectorParamsAs1DForOutWhenUnconnected=off
  Out2 : Outport  Port=2  InitialOutput=[0]  VectorParamsAs1DForOutWhenUnconnected=off
  Out3 : Outport  Port=3  InitialOutput=[0]  VectorParamsAs1DForOutWhenUnconnected=off
  wires:
  Delay1/1 -> Out3/1
  Delay/1 -> Out2/1
  In1/1 -> Out1/1, Delay1/1, Delay/1

== system VCM_main/Error display Box/Error Info/error memory MC4/Triggered Subsystem ==
  In1 : Inport
  Trigger : TriggerPort  VariantControl=Variant
  Delay : Delay  DelayLength=1  InitialCondition=0
  Delay1 : Delay  InitialCondition=0
  Out1 : Outport  VectorParamsAs1DForOutWhenUnconnected=off
  Out2 : Outport  Port=2  InitialOutput=[0]  VectorParamsAs1DForOutWhenUnconnected=off
  Out3 : Outport  Port=3  InitialOutput=[0]  VectorParamsAs1DForOutWhenUnconnected=off
  wires:
  Delay1/1 -> Out3/1
  Delay/1 -> Out2/1
  In1/1 -> Out1/1, Delay1/1, Delay/1

== system VCM_main/Error display Box/Error Info1/error memory MC1/Triggered Subsystem ==
  In1 : Inport
  Trigger : TriggerPort  VariantControl=Variant
  Delay : Delay  DelayLength=1  InitialCondition=0
  Delay1 : Delay  InitialCondition=0
  Out1 : Outport  VectorParamsAs1DForOutWhenUnconnected=off
  Out2 : Outport  Port=2  InitialOutput=[0]  VectorParamsAs1DForOutWhenUnconnected=off
  Out3 : Outport  Port=3  InitialOutput=[0]  VectorParamsAs1DForOutWhenUnconnected=off
  wires:
  Delay1/1 -> Out3/1
  Delay/1 -> Out2/1
  In1/1 -> Out1/1, Delay/1, Delay1/1

== system VCM_main/Error display Box/Error Info1/error memory MC2/Triggered Subsystem ==
  In1 : Inport
  Trigger : TriggerPort  VariantControl=Variant
  Delay : Delay  DelayLength=1  InitialCondition=0
  Delay1 : Delay  InitialCondition=0
  Out1 : Outport  VectorParamsAs1DForOutWhenUnconnected=off
  Out2 : Outport  Port=2  InitialOutput=[0]  VectorParamsAs1DForOutWhenUnconnected=off
  Out3 : Outport  Port=3  InitialOutput=[0]  VectorParamsAs1DForOutWhenUnconnected=off
  wires:
  Delay1/1 -> Out3/1
  Delay/1 -> Out2/1
  In1/1 -> Out1/1, Delay/1, Delay1/1

== system VCM_main/Error display Box/Error Info1/error memory MC3/Triggered Subsystem ==
  In1 : Inport
  Trigger : TriggerPort  VariantControl=Variant
  Delay : Delay  DelayLength=1  InitialCondition=0
  Delay1 : Delay  InitialCondition=0
  Out1 : Outport  VectorParamsAs1DForOutWhenUnconnected=off
  Out2 : Outport  Port=2  InitialOutput=[0]  VectorParamsAs1DForOutWhenUnconnected=off
  Out3 : Outport  Port=3  InitialOutput=[0]  VectorParamsAs1DForOutWhenUnconnected=off
  wires:
  Delay1/1 -> Out3/1
  Delay/1 -> Out2/1
  In1/1 -> Out1/1, Delay/1, Delay1/1

== system VCM_main/Error display Box/Error Info1/error memory MC4/Triggered Subsystem ==
  In1 : Inport
  Trigger : TriggerPort  VariantControl=Variant
  Delay : Delay  DelayLength=1  InitialCondition=0
  Delay1 : Delay  InitialCondition=0
  Out1 : Outport  VectorParamsAs1DForOutWhenUnconnected=off
  Out2 : Outport  Port=2  InitialOutput=[0]  VectorParamsAs1DForOutWhenUnconnected=off
  Out3 : Outport  Port=3  InitialOutput=[0]  VectorParamsAs1DForOutWhenUnconnected=off
  wires:
  Delay1/1 -> Out3/1
  Delay/1 -> Out2/1
  In1/1 -> Out1/1, Delay/1, Delay1/1

== system VCM_main/Error display Box/Error Info2/error memory MC1/Triggered Subsystem ==
  In1 : Inport
  Trigger : TriggerPort  VariantControl=Variant
  Delay : Delay  DelayLength=1  InitialCondition=0
  Delay1 : Delay  InitialCondition=0
  Out1 : Outport  VectorParamsAs1DForOutWhenUnconnected=off
  Out2 : Outport  Port=2  InitialOutput=[0]  VectorParamsAs1DForOutWhenUnconnected=off
  Out3 : Outport  Port=3  InitialOutput=[0]  VectorParamsAs1DForOutWhenUnconnected=off
  wires:
  Delay1/1 -> Out3/1
  Delay/1 -> Out2/1
  In1/1 -> Out1/1, Delay/1, Delay1/1

== system VCM_main/Error display Box/Error Info2/error memory MC2/Triggered Subsystem ==
  In1 : Inport
  Trigger : TriggerPort  VariantControl=Variant
  Delay : Delay  DelayLength=1  InitialCondition=0
  Delay1 : Delay  InitialCondition=0
  Out1 : Outport  VectorParamsAs1DForOutWhenUnconnected=off
  Out2 : Outport  Port=2  InitialOutput=[0]  VectorParamsAs1DForOutWhenUnconnected=off
  Out3 : Outport  Port=3  InitialOutput=[0]  VectorParamsAs1DForOutWhenUnconnected=off
  wires:
  Delay1/1 -> Out3/1
  Delay/1 -> Out2/1
  In1/1 -> Out1/1, Delay/1, Delay1/1

== system VCM_main/Error display Box/Error Info2/error memory MC3/Triggered Subsystem ==
  In1 : Inport
  Trigger : TriggerPort  VariantControl=Variant
  Delay : Delay  DelayLength=1  InitialCondition=0
  Delay1 : Delay  InitialCondition=0
  Out1 : Outport  VectorParamsAs1DForOutWhenUnconnected=off
  Out2 : Outport  Port=2  InitialOutput=[0]  VectorParamsAs1DForOutWhenUnconnected=off
  Out3 : Outport  Port=3  InitialOutput=[0]  VectorParamsAs1DForOutWhenUnconnected=off
  wires:
  Delay1/1 -> Out3/1
  Delay/1 -> Out2/1
  In1/1 -> Out1/1, Delay/1, Delay1/1

== system VCM_main/Error display Box/Error Info2/error memory MC4/Triggered Subsystem ==
  In1 : Inport
  Trigger : TriggerPort  VariantControl=Variant
  Delay : Delay  DelayLength=1  InitialCondition=0
  Delay1 : Delay  InitialCondition=0
  Out1 : Outport  VectorParamsAs1DForOutWhenUnconnected=off
  Out2 : Outport  Port=2  InitialOutput=[0]  VectorParamsAs1DForOutWhenUnconnected=off
  Out3 : Outport  Port=3  InitialOutput=[0]  VectorParamsAs1DForOutWhenUnconnected=off
  wires:
  Delay1/1 -> Out3/1
  Delay/1 -> Out2/1
  In1/1 -> Out1/1, Delay/1, Delay1/1

== system VCM_main/Error display Box/Error Info3/error memory MC1/Triggered Subsystem ==
  In1 : Inport
  Trigger : TriggerPort  VariantControl=Variant
  Delay : Delay  DelayLength=1  InitialCondition=0
  Delay1 : Delay  InitialCondition=0
  Out1 : Outport  VectorParamsAs1DForOutWhenUnconnected=off
  Out2 : Outport  Port=2  InitialOutput=[0]  VectorParamsAs1DForOutWhenUnconnected=off
  Out3 : Outport  Port=3  InitialOutput=[0]  VectorParamsAs1DForOutWhenUnconnected=off
  wires:
  Delay1/1 -> Out3/1
  Delay/1 -> Out2/1
  In1/1 -> Out1/1, Delay/1, Delay1/1

== system VCM_main/Error display Box/Error Info3/error memory MC2/Triggered Subsystem ==
  In1 : Inport
  Trigger : TriggerPort  VariantControl=Variant
  Delay : Delay  DelayLength=1  InitialCondition=0
  Delay1 : Delay  InitialCondition=0
  Out1 : Outport  VectorParamsAs1DForOutWhenUnconnected=off
  Out2 : Outport  Port=2  InitialOutput=[0]  VectorParamsAs1DForOutWhenUnconnected=off
  Out3 : Outport  Port=3  InitialOutput=[0]  VectorParamsAs1DForOutWhenUnconnected=off
  wires:
  Delay1/1 -> Out3/1
  Delay/1 -> Out2/1
  In1/1 -> Out1/1, Delay/1, Delay1/1

== system VCM_main/Error display Box/Error Info3/error memory MC3/Triggered Subsystem ==
  In1 : Inport
  Trigger : TriggerPort  VariantControl=Variant
  Delay : Delay  DelayLength=1  InitialCondition=0
  Delay1 : Delay  InitialCondition=0
  Out1 : Outport  VectorParamsAs1DForOutWhenUnconnected=off
  Out2 : Outport  Port=2  InitialOutput=[0]  VectorParamsAs1DForOutWhenUnconnected=off
  Out3 : Outport  Port=3  InitialOutput=[0]  VectorParamsAs1DForOutWhenUnconnected=off
  wires:
  Delay1/1 -> Out3/1
  Delay/1 -> Out2/1
  In1/1 -> Out1/1, Delay/1, Delay1/1

== system VCM_main/Error display Box/Error Info3/error memory MC4/Triggered Subsystem ==
  In1 : Inport
  Trigger : TriggerPort  VariantControl=Variant
  Delay : Delay  DelayLength=1  InitialCondition=0
  Delay1 : Delay  InitialCondition=0
  Out1 : Outport  VectorParamsAs1DForOutWhenUnconnected=off
  Out2 : Outport  Port=2  InitialOutput=[0]  VectorParamsAs1DForOutWhenUnconnected=off
  Out3 : Outport  Port=3  InitialOutput=[0]  VectorParamsAs1DForOutWhenUnconnected=off
  wires:
  Delay1/1 -> Out3/1
  Delay/1 -> Out2/1
  In1/1 -> Out1/1, Delay/1, Delay1/1

== system VCM_main/VDC/80kw_limitation/Power Limit_1/FL Power Culc ==
  FL Torque : Inport
  FL Actual Speed : Inport  Port=2
  2-D Lookup Table : Lookup_n-D  BreakpointsForDimension1="[1.3000    2.7000    5.4000    7.9000   10.4000   12.5000   14.4000   16.0000   17.4000   18.5000   19.6000]"  BreakpointsForDimension2="[ 500        1000        2000        3000        4000        6000       10000       12000       15000       19000]"  Table=|  InternalRulePriority=Speed  RndMeth=Simplest  InputSameDT=on
      | [ 0.6437    0.7133    0.7364    0.7470    0.7543    0.7657    0.7700    0.7708    0.7756    0.7814
      |     0.5842    0.7048    0.7757    0.8040    0.8201    0.8392    0.8516    0.8544    0.8597    0.8650
      |     0.4494    0.6081    0.7335    0.7882    0.8194    0.8543    0.8820    0.8888    0.8971    0.9044
      |     0.3559    0.5190    0.6702    0.7426    0.7854    0.8342    0.8758    0.8865    0.8984    0.9086
      |     0.2914    0.4478    0.6101    0.6941    0.7457    0.8062    0.8593    0.8758    0.8886    0.9016
      |     0.2417    0.3871    0.5522    0.6439    0.7024    0.7730    0.8373    0.8548    0.8737    0.8898
      |     0.2041    0.3371    0.5004    0.5965    0.6599    0.7388    0.8133    0.8342    0.8566    0.8759
      |     0.1731    0.2940    0.4510    0.5487    0.6155    0.7010    0.7856    0.8097    0.8356    0.8581
      |     0.1482    0.2575    0.4067    0.5041    0.5728    0.6634    0.7570    0.7840    0.8134    0.8271
      |     0.1281    0.2267    0.3672    0.4630    0.5325    0.6267    0.7277    0.7575    0.7902    0.7696
      |     0.1117    0.2005    0.3321    0.4251    0.4944    0.5909    0.6982    0.7306    0.6766    0.6928]
      settings: InputPortMap=u0,u1
  Divide : Product  Inputs=*/
  Gain : Gain  Gain=2*pi/60
  Product : Product
  Saturation : Saturate  UpperLimit=21  LowerLimit=0
  Saturation1 : Saturate  UpperLimit=19000  LowerLimit=0
  FL Power Consumption : Outport  VectorParamsAs1DForOutWhenUnconnected=off
  wires:
  Saturation1/1 -> Product/2, 2-D Lookup Table/2
  Saturation/1 -> Product/1, 2-D Lookup Table/1
  2-D Lookup Table/1 -> Divide/2  "FL Efficency"
  Product/1 -> Gain/1  "FL Motor Power"
  Divide/1 -> FL Power Consumption/1  "FL Power Consumption"
  FL Actual Speed/1 -> Saturation1/1
  FL Torque/1 -> Saturation/1
  Gain/1 -> Divide/1  "FL Motor Power_W"

== system VCM_main/VDC/80kw_limitation/Power Limit_1/FR Power Culc ==
  FR Torque : Inport
  FR Actual Speed : Inport  Port=2
  2-D Lookup Table : Lookup_n-D  BreakpointsForDimension1="[1.3000    2.7000    5.4000    7.9000   10.4000   12.5000   14.4000   16.0000   17.4000   18.5000   19.6000]"  BreakpointsForDimension2="[ 500        1000        2000        3000        4000        6000       10000       12000       15000       19000]"  Table=|  InternalRulePriority=Speed  RndMeth=Simplest  InputSameDT=on
      | [ 0.6437    0.7133    0.7364    0.7470    0.7543    0.7657    0.7700    0.7708    0.7756    0.7814
      |     0.5842    0.7048    0.7757    0.8040    0.8201    0.8392    0.8516    0.8544    0.8597    0.8650
      |     0.4494    0.6081    0.7335    0.7882    0.8194    0.8543    0.8820    0.8888    0.8971    0.9044
      |     0.3559    0.5190    0.6702    0.7426    0.7854    0.8342    0.8758    0.8865    0.8984    0.9086
      |     0.2914    0.4478    0.6101    0.6941    0.7457    0.8062    0.8593    0.8758    0.8886    0.9016
      |     0.2417    0.3871    0.5522    0.6439    0.7024    0.7730    0.8373    0.8548    0.8737    0.8898
      |     0.2041    0.3371    0.5004    0.5965    0.6599    0.7388    0.8133    0.8342    0.8566    0.8759
      |     0.1731    0.2940    0.4510    0.5487    0.6155    0.7010    0.7856    0.8097    0.8356    0.8581
      |     0.1482    0.2575    0.4067    0.5041    0.5728    0.6634    0.7570    0.7840    0.8134    0.8271
      |     0.1281    0.2267    0.3672    0.4630    0.5325    0.6267    0.7277    0.7575    0.7902    0.7696
      |     0.1117    0.2005    0.3321    0.4251    0.4944    0.5909    0.6982    0.7306    0.6766    0.6928]
      settings: InputPortMap=u0,u1
  Divide : Product  Inputs=*/
  Gain : Gain  Gain=2*pi/60
  Product : Product
  Saturation : Saturate  UpperLimit=21  LowerLimit=0
  Saturation1 : Saturate  UpperLimit=19000  LowerLimit=0
  Scope : Scope
  FR Power Consumption : Outport  VectorParamsAs1DForOutWhenUnconnected=off
  wires:
  Saturation1/1 -> Product/2, 2-D Lookup Table/2
  Saturation/1 -> Product/1, 2-D Lookup Table/1
  2-D Lookup Table/1 -> Divide/2  "FR Efficency"
  Product/1 -> Gain/1  "FR Motor Power"
  Divide/1 -> FR Power Consumption/1  "FR Power Consumption"
  FR Actual Speed/1 -> Saturation1/1
  FR Torque/1 -> Saturation/1
  Gain/1 -> Divide/1, Scope/1  "FR Motor Power_W"

== system VCM_main/VDC/80kw_limitation/Power Limit_1/RL Power Culc ==
  RL Torque : Inport
  RL Actual Speed : Inport  Port=2
  2-D Lookup Table : Lookup_n-D  BreakpointsForDimension1="[1.3000    2.7000    5.4000    7.9000   10.4000   12.5000   14.4000   16.0000   17.4000   18.5000   19.6000]"  BreakpointsForDimension2="[ 500        1000        2000        3000        4000        6000       10000       12000       15000       19000]"  Table=|  InternalRulePriority=Speed  RndMeth=Simplest  InputSameDT=on
      | [ 0.6437    0.7133    0.7364    0.7470    0.7543    0.7657    0.7700    0.7708    0.7756    0.7814
      |     0.5842    0.7048    0.7757    0.8040    0.8201    0.8392    0.8516    0.8544    0.8597    0.8650
      |     0.4494    0.6081    0.7335    0.7882    0.8194    0.8543    0.8820    0.8888    0.8971    0.9044
      |     0.3559    0.5190    0.6702    0.7426    0.7854    0.8342    0.8758    0.8865    0.8984    0.9086
      |     0.2914    0.4478    0.6101    0.6941    0.7457    0.8062    0.8593    0.8758    0.8886    0.9016
      |     0.2417    0.3871    0.5522    0.6439    0.7024    0.7730    0.8373    0.8548    0.8737    0.8898
      |     0.2041    0.3371    0.5004    0.5965    0.6599    0.7388    0.8133    0.8342    0.8566    0.8759
      |     0.1731    0.2940    0.4510    0.5487    0.6155    0.7010    0.7856    0.8097    0.8356    0.8581
      |     0.1482    0.2575    0.4067    0.5041    0.5728    0.6634    0.7570    0.7840    0.8134    0.8271
      |     0.1281    0.2267    0.3672    0.4630    0.5325    0.6267    0.7277    0.7575    0.7902    0.7696
      |     0.1117    0.2005    0.3321    0.4251    0.4944    0.5909    0.6982    0.7306    0.6766    0.6928]
      settings: InputPortMap=u0,u1
  Divide : Product  Inputs=*/
  Gain : Gain  Gain=2*pi/60
  Product : Product
  Saturation : Saturate  UpperLimit=21  LowerLimit=0
  Saturation1 : Saturate  UpperLimit=19000  LowerLimit=0
  RL Power Consumption : Outport  VectorParamsAs1DForOutWhenUnconnected=off
  wires:
  Saturation1/1 -> Product/2, 2-D Lookup Table/2
  Saturation/1 -> Product/1, 2-D Lookup Table/1
  2-D Lookup Table/1 -> Divide/2  "RL Efficency"
  Product/1 -> Gain/1  "RL Motor Power"
  Divide/1 -> RL Power Consumption/1  "RL Power Consumption"
  RL Actual Speed/1 -> Saturation1/1
  RL Torque/1 -> Saturation/1
  Gain/1 -> Divide/1  "RL Motor Power_W"

== system VCM_main/VDC/80kw_limitation/Power Limit_1/RR Power Culc ==
  RR Torque : Inport
  RR Actual Speed : Inport  Port=2
  2-D Lookup Table : Lookup_n-D  BreakpointsForDimension1="[1.3000    2.7000    5.4000    7.9000   10.4000   12.5000   14.4000   16.0000   17.4000   18.5000   19.6000]"  BreakpointsForDimension2="[ 500        1000        2000        3000        4000        6000       10000       12000       15000       19000]"  Table=|  InternalRulePriority=Speed  RndMeth=Simplest  InputSameDT=on
      | [ 0.6437    0.7133    0.7364    0.7470    0.7543    0.7657    0.7700    0.7708    0.7756    0.7814
      |     0.5842    0.7048    0.7757    0.8040    0.8201    0.8392    0.8516    0.8544    0.8597    0.8650
      |     0.4494    0.6081    0.7335    0.7882    0.8194    0.8543    0.8820    0.8888    0.8971    0.9044
      |     0.3559    0.5190    0.6702    0.7426    0.7854    0.8342    0.8758    0.8865    0.8984    0.9086
      |     0.2914    0.4478    0.6101    0.6941    0.7457    0.8062    0.8593    0.8758    0.8886    0.9016
      |     0.2417    0.3871    0.5522    0.6439    0.7024    0.7730    0.8373    0.8548    0.8737    0.8898
      |     0.2041    0.3371    0.5004    0.5965    0.6599    0.7388    0.8133    0.8342    0.8566    0.8759
      |     0.1731    0.2940    0.4510    0.5487    0.6155    0.7010    0.7856    0.8097    0.8356    0.8581
      |     0.1482    0.2575    0.4067    0.5041    0.5728    0.6634    0.7570    0.7840    0.8134    0.8271
      |     0.1281    0.2267    0.3672    0.4630    0.5325    0.6267    0.7277    0.7575    0.7902    0.7696
      |     0.1117    0.2005    0.3321    0.4251    0.4944    0.5909    0.6982    0.7306    0.6766    0.6928]
      settings: InputPortMap=u0,u1
  Divide : Product  Inputs=*/
  Gain : Gain  Gain=2*pi/60
  Product : Product
  Saturation : Saturate  UpperLimit=21  LowerLimit=0
  Saturation1 : Saturate  UpperLimit=19000  LowerLimit=0
  RR Power Consumption : Outport  VectorParamsAs1DForOutWhenUnconnected=off
  wires:
  Saturation1/1 -> Product/2, 2-D Lookup Table/2
  Saturation/1 -> Product/1, 2-D Lookup Table/1
  2-D Lookup Table/1 -> Divide/2  "RR Efficency"
  Product/1 -> Gain/1  "RR Motor Power"
  Divide/1 -> RR Power Consumption/1  "RR Power Consumption"
  RR Actual Speed/1 -> Saturation1/1
  RR Torque/1 -> Saturation/1
  Gain/1 -> Divide/1  "RR Motor Power_W"
